simulink model "A1_v1"  (R2023b)
settings: Solver=FixedStepAuto  StartTime=0.0  StopTime=10.0  FixedStep=1e-3  RelTol=1e-3  EnableMultiTasking=on
undefined symbols (not defined in the file): D0, D1, D10, D11, D12, D13, D2, D3, D4, D5, D6, D7, D8, D9, PTA0, PTA1, PTA2, PTB23, PTB9, PTC16, PTC17, PTC2, PTC3, PTC4, PTD0, PTD1, PTD2, PTD3
libraries: frdmk64flib x14
settings Model: ExtModeTrigDuration=5  Creator=Bernic  LastModifiedBy=cheni
settings SolverCC: AlgebraicLoopSolver=TrustRegion
settings OptimizationCC: EnhancedBackFolding=on  PassReuseOutputArgsAs=Individual arguments  ZeroExternalMemoryAtStartup=off  ZeroInternalMemoryAtStartup=off  MaxStackSize=64  OptimizeBlockOrder=speed  DifferentSizesBufferReuse=on  OptimizationCustomize=off  EfficientTunableParamExpr=on
settings DebuggingCC: ParameterTunabilityLossMsg=error
settings HardwareCC: ProdBitPerPointer=32  ProdBitPerSizeT=32  ProdBitPerPtrDiffT=32  ProdLargestAtomicInteger=Long  ProdLargestAtomicFloat=Double  ProdWordSize=32  ProdHWDeviceType=ARM Compatible->ARM Cortex
settings SFSimCC: MATLABDynamicMemAlloc=off
settings RTWCC: Description=Embedded Coder  SystemTargetFile=ert.tlc  HardwareBoard=NXP FRDM-K64F  TLCOptions="-aInlineSetEventsForThisBaseRateFcn=TLC_FALSE -aSuppressMultiTaskScheduler=TLC_FALSE  -aRateBasedStepFcn=0"  TemplateMakefile=ert_default_tmf  Toolchain=GNU Tools for ARM Embedded Processors
settings CodeAppCC: ForceParamTrailComments=on  IgnoreCustomStorageClasses=off  OperatorAnnotations=on  SimulinkDataObjDesc=on  SFDataObjDesc=on  InsertBlockDesc=on
settings ERTTargetCC: ExtModeTransport=4  ExtModeMexFile=sendToCommService

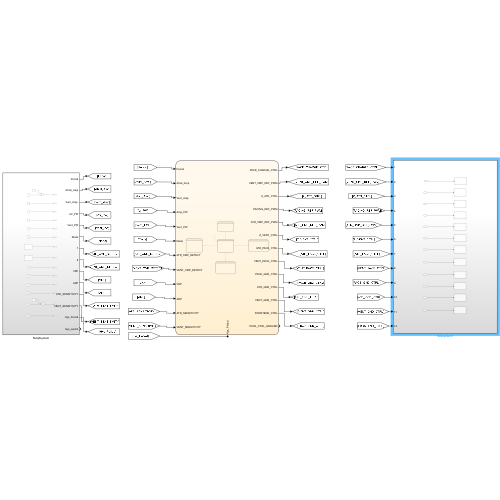
[thumbnail: Simulink's stored preview of the top-level diagram]
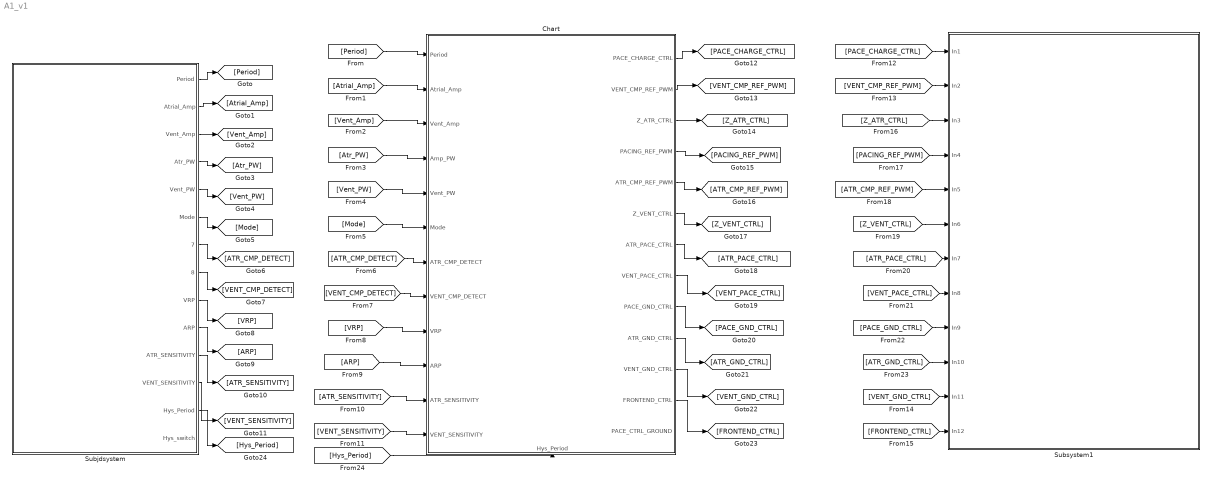
== system A1_v1 ==
  Chart : Stateflow chart  TreatAsAtomicUnit=on
      settings: PortSchema="{\"entries\":[{\"content\":{\"sides\":[{\"content\":{\"connectorIds\":[\"In6\",\"In2\",\"In3\",\"In4\",\"In5\",\"In7\",\"In8\",\"In9\",\"In10\",\"In11\",\"In12\",\"In13\"]},\"type\":\"ConnectorPlacement.EquallySpacedRectSide\",\"uuid\":\"6343ef83-1ce8-46c7-8622-1dca0f09a909\"},{\"content\":{\"connectorIds\":[\"Out1\",\"Out2\",\"Out3\",\"Out4\",\"Out5\",\"Out6\",\"Out7\",\"Out8\",\"Out9\",\"Out10\",\"Out11\",\"Out12\",\"Out13\"],\"side\":\"RIGHT\"},\"type\":\"ConnectorPlacement.EquallySpacedRectSide\",\"uuid\":\"7d8c9973-a2ea-42d1-99a2-efee47476445\"},{\"content\":{\"side\":\"TOP\"},\"type\":\"ConnectorPlacement.EquallySpacedRectSide\",\"uuid\":\"d6f36041-fe62-4fd0-b92e-ddcbd2ff161d\"},{\"content\":{\"connectorIds\":[\"In1\"],\"side\":\"BOTTOM\"},\"type\":\"ConnectorPlacement.EquallySpacedRectSide\",\"uuid\":\"9ef693f9-8331-444a-9668-ba4dbf8aea62\"}]},\"type\":\"ConnectorPlacement.EquallySpacedConnector\",\"uuid\":\"1488a652-70a0-4b94-9610-167d4f46302b\"}],\"packageUris\":[\"http://schema.mathworks.com/mf0/Connector/R2020b\"],\"version\":\"1.0\"}"
  Subjdsystem : Subsystem
  Subsystem1 : Subsystem
  wires:
  Subjdsystem/1(Period) -> [Period]
  Subjdsystem/2(Atrial_Amp) -> [Atrial_Amp]
  Subjdsystem/3("Vent_Amp ") -> [Vent_Amp]
  Subjdsystem/4(Atr_PW) -> [Atr_PW]
  Subjdsystem/5(Vent_PW) -> [Vent_PW]
  Subjdsystem/6(Mode) -> [Mode]
  [Period] -> Chart/6(Period)
  [Atrial_Amp] -> Chart/2(Atrial_Amp)
  [Vent_Amp] -> Chart/3(Vent_Amp)
  [Atr_PW] -> Chart/4(Amp_PW)
  [Vent_PW] -> Chart/5(Vent_PW)
  [Mode] -> Chart/7(Mode)
  Subjdsystem/7(7) -> [ATR_CMP_DETECT]
  Subjdsystem/8(8) -> [VENT_CMP_DETECT]
  Subjdsystem/9(VRP) -> [VRP]
  Subjdsystem/10(ARP) -> [ARP]
  Subjdsystem/11(ATR_SENSITIVITY) -> [ATR_SENSITIVITY]
  Subjdsystem/12(VENT_SENSITIVITY) -> [VENT_SENSITIVITY]
  [ATR_CMP_DETECT] -> Chart/8(ATR_CMP_DETECT)
  [VENT_CMP_DETECT] -> Chart/9(VENT_CMP_DETECT)
  [VRP] -> Chart/10(VRP)
  [ARP] -> Chart/11(ARP)
  [ATR_SENSITIVITY] -> Chart/12(ATR_SENSITIVITY)
  [VENT_SENSITIVITY] -> Chart/13(VENT_SENSITIVITY)
  [PACE_CHARGE_CTRL] -> Subsystem1/1(In1)
  [VENT_CMP_REF_PWM] -> Subsystem1/2(In2)
  [Z_ATR_CTRL] -> Subsystem1/3(In3)
  [PACING_REF_PWM] -> Subsystem1/4(In4)
  [ATR_CMP_REF_PWM] -> Subsystem1/5(In5)
  [Z_VENT_CTRL] -> Subsystem1/6(In6)
  [ATR_PACE_CTRL] -> Subsystem1/7(In7)
  [VENT_PACE_CTRL] -> Subsystem1/8(In8)
  [PACE_GND_CTRL] -> Subsystem1/9(In9)
  [ATR_GND_CTRL] -> Subsystem1/10(In10)
  [VENT_GND_CTRL] -> Subsystem1/11(In11)
  [FRONTEND_CTRL] -> Subsystem1/12(In12)
  Chart/1(PACE_CHARGE_CTRL) -> [PACE_CHARGE_CTRL]
  Chart/2(VENT_CMP_REF_PWM) -> [VENT_CMP_REF_PWM]
  Chart/3(Z_ATR_CTRL) -> [Z_ATR_CTRL]
  Chart/4(PACING_REF_PWM) -> [PACING_REF_PWM]
  Chart/5(ATR_CMP_REF_PWM) -> [ATR_CMP_REF_PWM]
  Chart/6(Z_VENT_CTRL) -> [Z_VENT_CTRL]
  Chart/7(ATR_PACE_CTRL) -> [ATR_PACE_CTRL]
  Chart/8(VENT_PACE_CTRL) -> [VENT_PACE_CTRL]
  Chart/9(PACE_GND_CTRL) -> [PACE_GND_CTRL]
  Chart/10(ATR_GND_CTRL) -> [ATR_GND_CTRL]
  Chart/11(VENT_GND_CTRL) -> [VENT_GND_CTRL]
  Chart/12(FRONTEND_CTRL) -> [FRONTEND_CTRL]
  Subjdsystem/13(Hys_Period) -> [Hys_Period]
  [Hys_Period] -> Chart/1(Hys_Period)

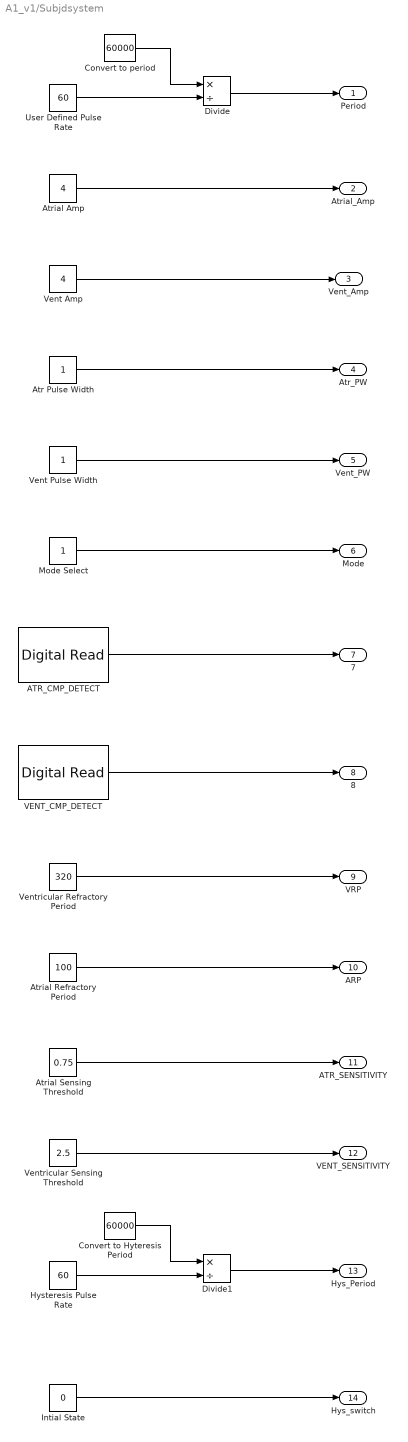
== system A1_v1/Subjdsystem ==
  ATR_CMP_DETECT : frdmk64flib/Digital Read  Whichpin=PTC16 (D0)  SampleTime=-1
  Atr Pulse Width : Constant
  Atrial Amp : Constant  Value=4
  Atrial Refractory Period : Constant  Value=100  VectorParams1D=off
  Atrial Sensing Threshold : Constant  Value=0.75  VectorParams1D=off
  Convert to Hyteresis Period : Constant  Value=60000  VectorParams1D=off
  Convert to period : Constant  Value=60000  VectorParams1D=off
  Divide : Product  Inputs=*/
  Divide1 : Product  Inputs=*/
  Hysteresis Pulse Rate : Constant  Value=60  VectorParams1D=off
  Intial State : Constant  Value=0  VectorParams1D=off
  Mode Select : Constant  VectorParams1D=off
  User Defined Pulse Rate : Constant  Value=60  VectorParams1D=off
  VENT_CMP_DETECT : frdmk64flib/Digital Read  Whichpin=PTC17 (D1)  SampleTime=-1
  Vent Amp : Constant  Value=4
  Vent Pulse Width : Constant  VectorParams1D=off
  Ventricular Refractory Period : Constant  Value=320  VectorParams1D=off
  Ventricular Sensing Threshold : Constant  Value=2.5  VectorParams1D=off
  Period : Outport
  Atrial_Amp : Outport  Port=2
  "Vent_Amp " : Outport  Port=3
  Atr_PW : Outport  Port=4
  Vent_PW : Outport  Port=5
  Mode : Outport  Port=6
  7 : Outport  Port=7
  8 : Outport  Port=8
  VRP : Outport  Port=9
  ARP : Outport  Port=10
  ATR_SENSITIVITY : Outport  Port=11
  VENT_SENSITIVITY : Outport  Port=12
  Hys_Period : Outport  Port=13
  Hys_switch : Outport  Port=14
  wires:
  User Defined Pulse Rate/1 -> Divide/2
  Atrial Amp/1 -> Atrial_Amp/1
  Vent Amp/1 -> "Vent_Amp "/1
  Atr Pulse Width/1 -> Atr_PW/1
  Vent Pulse Width/1 -> Vent_PW/1
  Divide/1 -> Period/1
  Convert to period/1 -> Divide/1
  Mode Select/1 -> Mode/1
  ATR_CMP_DETECT/1 -> 7/1
  VENT_CMP_DETECT/1 -> 8/1
  Atrial Refractory Period/1 -> ARP/1
  Ventricular Refractory Period/1 -> VRP/1
  Atrial Sensing Threshold/1 -> ATR_SENSITIVITY/1
  Ventricular Sensing Threshold/1 -> VENT_SENSITIVITY/1
  Convert to Hyteresis Period/1 -> Divide1/1
  Divide1/1 -> Hys_Period/1
  Hysteresis Pulse Rate/1 -> Divide1/2
  Intial State/1 -> Hys_switch/1

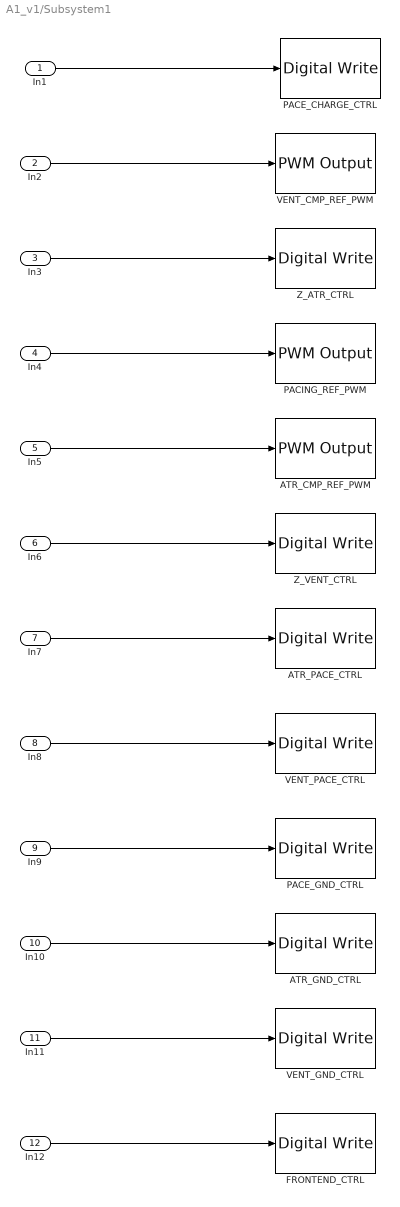
== system A1_v1/Subsystem1 ==
  In1 : Inport
  In2 : Inport  Port=2
  In3 : Inport  Port=3
  In4 : Inport  Port=4
  In5 : Inport  Port=5
  In6 : Inport  Port=6
  In7 : Inport  Port=7
  In8 : Inport  Port=8
  In9 : Inport  Port=9
  In10 : Inport  Port=10
  In11 : Inport  Port=11
  In12 : Inport  Port=12
  ATR_CMP_REF_PWM : frdmk64flib/PWM Output  Whichpin=PTC2 (D6)  InitialFrequency=2000  InitialDutyCycle=0
  ATR_GND_CTRL : frdmk64flib/Digital Write  Whichpin=PTD2 (D11)
  "ATR_PACE_CTRL " : frdmk64flib/Digital Write  Whichpin=PTA0 (D8)
  FRONTEND_CTRL : frdmk64flib/Digital Write  Whichpin=PTD1 (D13)
  PACE_CHARGE_CTRL : frdmk64flib/Digital Write  Whichpin=PTB9 (D2)
  "PACE_GND_CTRL " : frdmk64flib/Digital Write  Whichpin=PTD0 (D10)
  PACING_REF_PWM : frdmk64flib/PWM Output  Whichpin=PTA2 (D5)  InitialFrequency=2000  InitialDutyCycle=0
  VENT_CMP_REF_PWM : frdmk64flib/PWM Output  Whichpin=PTA1 (D3)  InitialFrequency=2000  InitialDutyCycle=0
  "VENT_GND_CTRL " : frdmk64flib/Digital Write  Whichpin=PTD3 (D12)
  VENT_PACE_CTRL : frdmk64flib/Digital Write  Whichpin=PTC4 (D9)
  Z_ATR_CTRL : frdmk64flib/Digital Write  Whichpin=PTB23 (D4)
  Z_VENT_CTRL : frdmk64flib/Digital Write  Whichpin=PTC3 (D7)
  wires:
  In1/1 -> PACE_CHARGE_CTRL/1
  In2/1 -> VENT_CMP_REF_PWM/1
  In3/1 -> Z_ATR_CTRL/1
  In4/1 -> PACING_REF_PWM/1
  In5/1 -> ATR_CMP_REF_PWM/1
  In6/1 -> Z_VENT_CTRL/1
  In7/1 -> "ATR_PACE_CTRL "/1
  In8/1 -> VENT_PACE_CTRL/1
  In12/1 -> FRONTEND_CTRL/1
  In9/1 -> "PACE_GND_CTRL "/1
  In11/1 -> "VENT_GND_CTRL "/1
  In10/1 -> ATR_GND_CTRL/1

== stateflow chart A1_v1/Chart ==
  state VOO
    state Charging
      entry:
      %Charging C22
      ATR_PACE_CTRL = 0
      VENT_PACE_CTRL = 0
      PACING_REF_PWM = Vent_Amp
      PACE_CHARGE_CTRL = 1
      %Discharging C21
      PACE_CTRL_GROUND = 1
      VENT_PACE_CTRL = 0
      Z_ATR_CTRL = 0
      Z_VENT_CTRL = 0
      ATR_PACE_CTRL = 0
      ATR_GND_CTRL = 0
      VENT_GND_CTRL = 1
    state Discharging
      entry:
      %Discharge C22 into C21
      PACE_CHARGE_CTRL = 0
      PACE_GND_CTRL = 1
      ATR_PACE_CTRL = 0
      ATR_GND_CTRL = 0
      Z_VENT_CTRL = 0
      Z_ATR_CTRL = 0
      VENT_GND_CTRL = 0
      VENT_PACE_CTRL = 1
    (default) -> VOO.Charging
    VOO.Charging -> Discharging : [[after(Vent_PW, msec)]]
    Discharging -> VOO.Charging : [[after(Period - Vent_PW, msec)]]
  state AAI
    state Hys_start
      Hys=1
    state Pacing
      entry:
      % Discharging C22 to C21
      PACE_CHARGE_CTRL = 0
      PACE_GND_CTRL = 1
      VENT_PACE_CTRL = 0
      Z_ATR_CTRL = 0
      Z_VENT_CTRL = 0
      ATR_PACE_CTRL = 1
      ATR_GND_CTRL = 0
      VENT_GND_CTRL = 0
    state Charging_sensing
      entry:
      %Sensing on
      FRONTEND_CTRL = 1
      ATR_CMP_REF_PWM = ATR_SENSITIVITY
      % Charging C22
      ATR_PACE_CTRL = 0
      VENT_PACE_CTRL = 0
      PACING_REF_PWM = Atrial_Amp
      PACE_CHARGE_CTRL = 1
      %  Discharge C21 while
      PACE_GND_CTRL = 1
      ATR_PACE_CTRL = 0
      Z_ATR_CTRL = 0
      Z_VENT_CTRL = 0
      ATR_GND_CTRL = 1
      VENT_GND_CTRL = 0
      VENT_PACE_CTRL = 0
    AAI.Hys_start -> AAI.Charging_sensing
    (junction 42) -> AAI.Hys_start [order 1] : [ATR_CMP_DETECT ==1]
    (default) -> AAI.Charging_sensing
    AAI.Charging_sensing -> (junction 42) : {after(ARP, msec)}
    (junction 42) -> AAI.Pacing [order 2] : [(Hys==0)&&(ATR_CMP_DETECT==0)] {after(Period - ARP - Atr_PW, msec)}
    (junction 42) -> AAI.Pacing [order 3] : [(Hys==1)&&(VENT_CMP_DETECT==0)] {after(Hys_Period-ARP-Atr_PW, msec)}
    AAI.Pacing -> AAI.Charging_sensing : {after(Atr_PW, msec)}
  state Mode_Start
  state AOO
    state Charging
      entry:
      % Charging C22
      ATR_PACE_CTRL = 0
      VENT_PACE_CTRL = 0
      PACING_REF_PWM = Atrial_Amp
      PACE_CHARGE_CTRL = 1
      %  Discharge C21 while
      PACE_GND_CTRL = 1
      ATR_PACE_CTRL = 0
      Z_ATR_CTRL = 0
      Z_VENT_CTRL = 0
      ATR_GND_CTRL = 1
      VENT_GND_CTRL = 0
      VENT_PACE_CTRL = 0
    state Pacing
      entry:
      % Discharging C22 to C21
      PACE_CHARGE_CTRL = 0
      PACE_GND_CTRL = 1
      VENT_PACE_CTRL = 0
      Z_ATR_CTRL = 0
      Z_VENT_CTRL = 0
      ATR_PACE_CTRL = 1
      ATR_GND_CTRL = 0
      VENT_GND_CTRL = 0
    (default) -> AOO.Charging
    AOO.Pacing -> AOO.Charging : [after(Atr_PW, msec)]
    AOO.Charging -> AOO.Pacing : [after(Period - Atr_PW, msec)]
  state VVI
    state Charging_sensing
      entry:
      %sensing
      FRONTEND_CTRL=1
      VENT_CMP_REF_PWM = VENT_SENSITIVITY
      % Charging C22
      ATR_PACE_CTRL = 0
      VENT_PACE_CTRL = 0
      PACING_REF_PWM = Vent_Amp
      PACE_CHARGE_CTRL = 1
      %  Discharge C21 while
      PACE_GND_CTRL = 1
      ATR_PACE_CTRL = 0
      Z_ATR_CTRL = 0
      Z_VENT_CTRL = 0
      ATR_GND_CTRL = 0
      VENT_GND_CTRL = 0
      VENT_PACE_CTRL = 0
    state Pacing
      entry:
      % Discharging C22 to C21
      PACE_CHARGE_CTRL = 0
      PACE_GND_CTRL = 1
      ATR_PACE_CTRL = 0
      Z_ATR_CTRL = 0
      Z_VENT_CTRL = 0
      ATR_PACE_CTRL = 0
      ATR_GND_CTRL = 0
      VENT_GND_CTRL = 1
    state Hys_start
      Hys=1
    (default) -> VVI.Charging_sensing
    VVI.Pacing -> VVI.Charging_sensing : {after(Vent_PW, msec)}
    (junction 106) -> VVI.Pacing [order 2] : [(Hys==0)&&(VENT_CMP_DETECT==0)]{after(Period-Vent_PW-VRP, msec)}
    VVI.Charging_sensing -> (junction 106) : {after(VRP, msec)}
    (junction 106) -> VVI.Pacing [order 3] : [(Hys==1)&&(VENT_CMP_DETECT==1)]{after(Hys_Period-Vent_PW-VRP, msec)}
    (junction 106) -> VVI.Hys_start [order 1] : [VENT_CMP_DETECT==1]
    VVI.Hys_start -> VVI.Charging_sensing
  Mode_Start -> VOO [order 1] : [Mode==1]
  (default) -> Mode_Start
  Mode_Start -> AAI [order 2] : [Mode==2]
  Mode_Start -> AOO [order 3] : [Mode==3]
  Mode_Start -> VVI [order 4] : [Mode==4]
  data: Hys_Period input; Atrial_Amp input; Vent_Amp input; Amp_PW input; Vent_PW input; Period input; Mode input; ATR_CMP_DETECT input; VENT_CMP_DETECT input; VRP input; ARP input; ATR_SENSITIVITY input; VENT_SENSITIVITY input; PACE_CHARGE_CTRL output; VENT_CMP_REF_PWM output; Z_ATR_CTRL output; PACING_REF_PWM output; ATR_CMP_REF_PWM output; Z_VENT_CTRL output; ATR_PACE_CTRL output; VENT_PACE_CTRL output; PACE_GND_CTRL output; ATR_GND_CTRL output; VENT_GND_CTRL output; FRONTEND_CTRL output; PACE_CTRL_GROUND output; Hys local; ATR_ constant double
